simulink model "Pi_MotionDetection_SAD"  (R2020b)
settings: Solver=FixedStepDiscrete  StartTime=0.0  StopTime=inf  RelTol=1e-3  EnableMultiTasking=on
undefined symbols (not defined in the file or in its folder): Rec, SDTV
libraries: visionanalysis x2, visionconversions x1, visiongeotforms x1, embdlinuxlib x1, dspvision x1, raspberrypiAVlib x1
settings Model: SimulationMode=external  ExtModeTrigDuration=100  Creator=The MathWorks, Inc.  LastModifiedBy=carlo
settings SolverCC: PositivePriorityOrder=on
settings DataIOCC: LimitDataPoints=on  SaveFormat=Array  ReturnWorkspaceOutputs=off
settings OptimizationCC: ExpressionDepthLimit=2147483647  LifeSpan=Inf  MaxStackSize=64
settings DebuggingCC: UnderspecifiedInitializationDetection=Classic  MergeDetectMultiDrivingBlocksExec=none  FcnCallInpInsideContextMsg=warning  AllowSymbolicDim=off  StateNameClashWarn=warning  SFUnexpectedBacktrackingDiag=warning  SFNoUnconditionalDefaultTransitionDiag=warning  SFExecutionAtInitializationDiag=none  ArithmeticOperatorsInVariantConditions=warning
settings HardwareCC: ProdBitPerPointer=32  ProdBitPerSizeT=32  ProdBitPerPtrDiffT=32  ProdLargestAtomicInteger=Long  ProdLargestAtomicFloat=Double  ProdWordSize=32  ProdHWDeviceType=ARM Compatible->ARM Cortex  UseEmbeddedCoderFeatures=off  UseSimulinkCoderFeatures=off
settings ModelReferenceCC: PropagateSignalLabelsOutOfModel=off
settings SFSimCC: SimUseLocalCustomCode=off  MATLABDynamicMemAlloc=off  CustomCodeUndefinedFunction=UseInterfaceOnly
settings RTWCC: Description=Embedded Coder  SystemTargetFile=ert.tlc  HardwareBoard=Raspberry Pi  TLCOptions=-aInlineSetEventsForThisBaseRateFcn=TLC_FALSE -aSuppressMultiTaskScheduler=TLC_FALSE -aRateBasedStepFcn=0  TemplateMakefile=ert_default_tmf  GenerateReport=on  RTWVerbose=off  RTWUseLocalCustomCode=off  Toolchain=GNU GCC Raspberry Pi  LaunchReport=on
settings CodeAppCC: ForceParamTrailComments=on  OperatorAnnotations=on  StateflowObjectComments=on  MATLABSourceComments=on
settings ERTTargetCC: MultiwordLength=2048  ERTCustomFileBanners=off  SupportContinuousTime=on  SupportNonInlinedSFcns=on  RemoveResetFunc=off  ModelStepFunctionPrototypeControlCompliant=off
settings ConfigComp: CovMetricSettings=dw  CovSaveCumulativeToWorkspaceVar=on  CovSaveSingleToWorkspaceVar=on  CovExternalEMLEnable=off

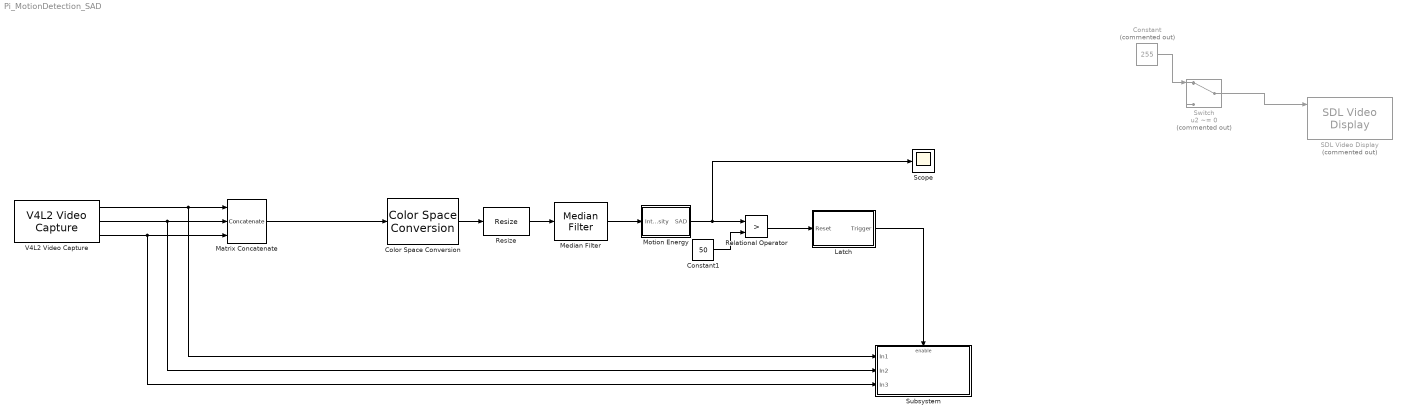
== system Pi_MotionDetection_SAD ==
  Color Space Conversion : visionconversions/Color Space  Conversion  conversion=Obsolete  conversionActive=R'G'B' to intensity  wp_str=D65  rec=Rec. 601 (SDTV)  sys=1125/60/2:1  imagePorts=One multidimensional signal
  Constant : Constant  Commented=on  Value=255  OutDataTypeStr=uint8
  Constant1 : Constant  Value=50  OutDataTypeStr=Inherit: Inherit via back propagation
  Latch : Subsystem
      mask Display: disp('Hold')
  Matrix Concatenate : Concatenate  NumInputs=3  Mode=Multidimensional array  ConcatenateDimension=3
  Median Filter : visionanalysis/Median Filter  nghbood=[3 3]  outSize=Same as input port I  padType=Symmetric  padSrc=Specify via dialog  padVal=0  roundingMode=Floor  overflowMode=off
      settings: SourceProductBaseCode=VP
  Motion Energy : Subsystem
  Relational Operator : RelationalOperator  Operator=>  OutDataTypeStr=boolean  RndMeth=Simplest
  Resize : visiongeotforms/Resize  specify=Output size as a percentage of input size  rfactor=[25 25]  outCols=25  outRows=25  outRowsCols=[240 320]  interp_method=Bilinear  antialias=on  useROI=off  roiFlag=off  roundingMode=Nearest  overflowMode=on  prodOutputMode=Binary point scaling  prodOutputWordLength=32  prodOutputFracLength=10
      settings: SourceProductBaseCode=VP
  SDL Video Display : embdlinuxlib/SDL Video Display  Commented=on  pixelFormat=RGB  pixelOrder=Planar  rowMajor=on  blockPlatform=Raspberry Pi
      settings: SourceProductBaseCode=SC_BEAGLEBONE_BLUE,NVIDIA,RASPPI
  Scope : Scope
  Subsystem : Subsystem
  Switch : Switch  Commented=on  Criteria=u2 ~= 0  Threshold=1
  V4L2 Video Capture : raspberrypiAVlib/V4L2 Video Capture  DeviceName=/dev/video0  Resolution=640x480  CustomResolution=[ 320, 240 ]  PixelFormat=RGB  SampleTime=1/24  pixelOrder=Planar  simOutput=Colorbars  imSizeSelection=320x240  imSize=[640, 480]  roi=[0, 0, 640, 480]  m_devName='/dev/video0'  blockPlatform=Raspberry Pi
      settings: SourceProductBaseCode=RASPPI
  wires:
  Median Filter/1 -> Motion Energy/1(Intensity)
  Constant/1 -> Switch/1
  Resize/1 -> Median Filter/1
  Motion Energy/1(SAD) -> Relational Operator/1, Scope/1
  Color Space Conversion/1 -> Resize/1
  V4L2 Video Capture/2 -> Subsystem/2(In2), Matrix Concatenate/2
  V4L2 Video Capture/1 -> Subsystem/1(In1), Matrix Concatenate/1
  V4L2 Video Capture/3 -> Subsystem/3(In3), Matrix Concatenate/3
  Switch/1 -> SDL Video Display/1
  Matrix Concatenate/1 -> Color Space Conversion/1
  Constant1/1 -> Relational Operator/2
  Relational Operator/1 -> Latch/1(Reset)
  Latch/1(Trigger) -> Subsystem/Enable

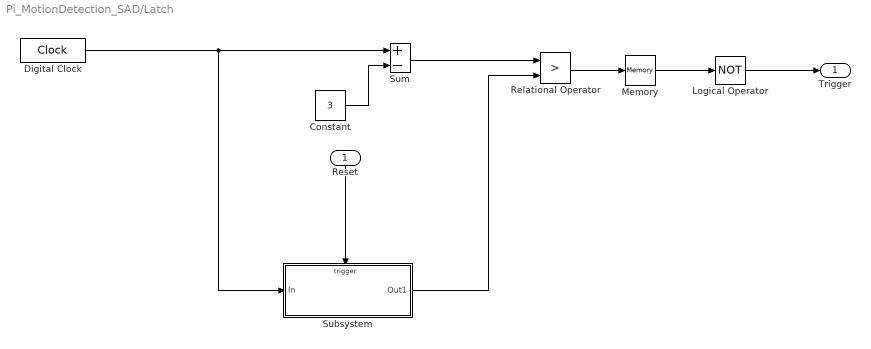
== system Pi_MotionDetection_SAD/Latch ==
  Reset : Inport
  Constant : Constant  Value=3
  Digital Clock : DigitalClock  SampleTime=-1
  Logical Operator : Logic  Operator=NOT  Inputs=1
  Memory : Memory  InitialCondition=1  InheritSampleTime=on
  Relational Operator : RelationalOperator  Operator=>  RndMeth=Nearest  InputSameDT=on
  Subsystem : Subsystem
  Sum : Sum  Inputs=+-  InputSameDT=on  SaturateOnIntegerOverflow=on  OutDataTypeStr=Inherit: Same as first input
  Trigger : Outport  InitialOutput=0  VectorParamsAs1DForOutWhenUnconnected=off
  wires:
  Reset/1 -> Subsystem/Trigger
  Sum/1 -> Relational Operator/1
  Subsystem/1(Out1) -> Relational Operator/2
  Relational Operator/1 -> Memory/1
  Memory/1 -> Logical Operator/1
  Logical Operator/1 -> Trigger/1
  Constant/1 -> Sum/2
  Digital Clock/1 -> Subsystem/1(In), Sum/1

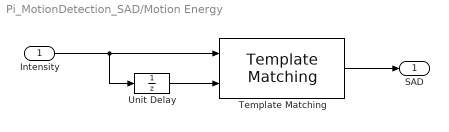
== system Pi_MotionDetection_SAD/Motion Energy ==
  Intensity : Inport
  Template Matching : visionanalysis/Template Matching  metric=Maximum absolute difference  output=Metric matrix  method=Exhaustive  nMetric=off  nSize=3  roi=off  roiValid=off  roundingMode=Floor  overflowMode=on  prodOutputMode=Binary point scaling  prodOutputWordLength=32  prodOutputFracLength=0
      settings: SourceProductBaseCode=VP
  Unit Delay : UnitDelay  SampleTime=-1  HasFrameUpgradeWarning=on
  SAD : Outport  VectorParamsAs1DForOutWhenUnconnected=off
  wires:
  Template Matching/1 -> SAD/1
  Intensity/1 -> Template Matching/1, Unit Delay/1
  Unit Delay/1 -> Template Matching/2

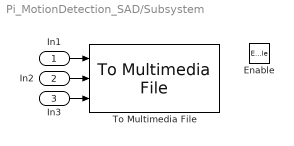
== system Pi_MotionDetection_SAD/Subsystem ==
  In1 : Inport
  In2 : Inport  Port=2
  In3 : Inport  Port=3
  Enable : EnablePort
  To Multimedia File : dspvision/To Multimedia File  outputFilename=output.avi  streamSelection=Video only  videoCompressor=None (uncompressed)  audioCompressor=None (uncompressed)  imagePorts=Separate color signals  fileType=AVI  audioDatatype=Determine from input data type  fourcc=RGB  videoQuality=75  mj2000CompFactor=10
  wires:
  In1/1 -> To Multimedia File/1
  In3/1 -> To Multimedia File/3
  In2/1 -> To Multimedia File/2

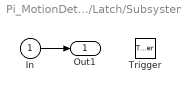
== system Pi_MotionDetection_SAD/Latch/Subsystem ==
  In : Inport
  Trigger : TriggerPort  TriggerType=either  VariantControl=Variant
  Out1 : Outport  InitialOutput=-10  VectorParamsAs1DForOutWhenUnconnected=off
  wires:
  In/1 -> Out1/1
